simulink model "DC_DC"  (R2020b)
settings: Solver=VariableStepAuto  StartTime=0.0  StopTime=0.1  RelTol=1e-3
libraries: powerlib x20, powerlib_meascontrol x1
settings Model: Creator=huang  LastModifiedBy=huang
settings SolverCC: ZeroCrossAlgorithm=Adaptive
settings DebuggingCC: IgnoredZcDiagnostic=none

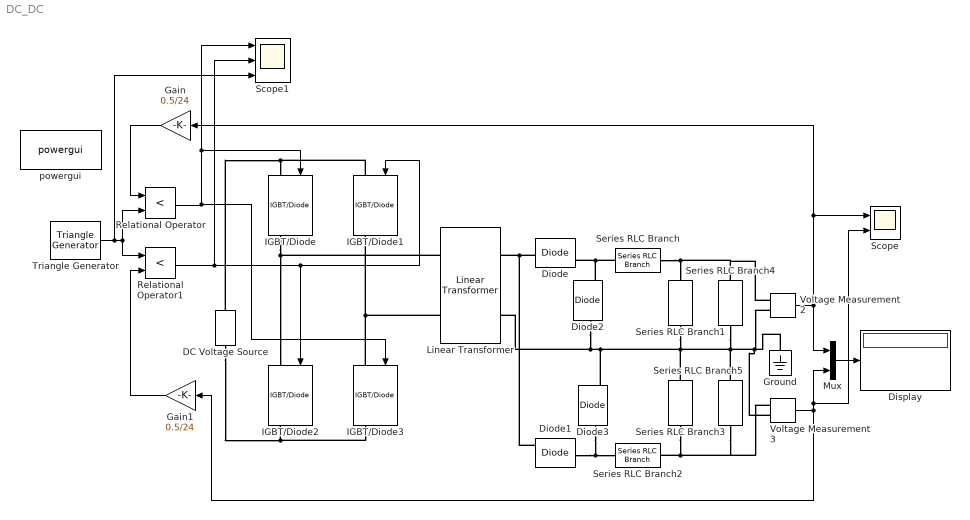
== system DC_DC ==
  DC Voltage Source : powerlib/Electrical Sources/DC Voltage Source  Amplitude=200  Measurements=None
  Diode{,1..3} (4 alike) : powerlib/Power Electronics/Diode  Ron=0.001  Lon=0  Vf=0.8  IC=0  UseSnubber=0  Rs=500  Cs=250e-9  Measurements=on
  Display : Display
  Gain : Gain  Gain=0.5/24
  Gain1 : Gain  Gain=0.5/24
  Ground : powerlib/Elements/Ground  LConnTagsString=a
  IGBT/Diode{,1..3} (4 alike) : powerlib/Power Electronics/IGBT//Diode  Ron=1e-3  Rs=1e5  Cs=inf  Measurements=on
  Linear Transformer : powerlib/Elements/Linear Transformer  UNITS=SI  NominalPower=[ 200 20e3 ]  winding1=[200 8e-08 5.0929e-11]  winding2=[48*2 2e-08 1.2732e-11]  ThreeWindings=off  winding3=[24*2 2e-08 1.2732e-11]  RmLm=[0.020001 3.1831e-07]  Measurements=None  DataType=on
  Mux : Mux  Inputs=2
  Relational Operator : RelationalOperator  Operator=<  OutDataTypeStr=boolean  RndMeth=Simplest
  Relational Operator1 : RelationalOperator  Operator=<  OutDataTypeStr=boolean  RndMeth=Simplest
  Scope : Scope  NumInputPorts=2
  Scope1 : Scope  NumInputPorts=3
  Series RLC Branch : powerlib/Elements/Series RLC Branch  LConnTagsString=__new0  RConnTagsString=__new0  BranchType=L  Resistance=1  Inductance=2e-3  SetiL0=off  InitialCurrent=0  Capacitance=1e-6  Setx0=off  InitialVoltage=0  Measurements=None
  Series RLC Branch1 : powerlib/Elements/Series RLC Branch  LConnTagsString=__new0  RConnTagsString=__new0  BranchType=C  Resistance=1  Inductance=1e-3  SetiL0=off  InitialCurrent=0  Capacitance=100e-6  Setx0=off  InitialVoltage=0  Measurements=None
  Series RLC Branch2 : powerlib/Elements/Series RLC Branch  LConnTagsString=__new0  RConnTagsString=__new0  BranchType=L  Resistance=1  Inductance=2e-3  SetiL0=off  InitialCurrent=0  Capacitance=1e-6  Setx0=off  InitialVoltage=0  Measurements=None
  Series RLC Branch3 : powerlib/Elements/Series RLC Branch  LConnTagsString=__new0  RConnTagsString=__new0  BranchType=C  Resistance=1  Inductance=1e-3  SetiL0=off  InitialCurrent=0  Capacitance=100e-6  Setx0=off  InitialVoltage=0  Measurements=None
  Series RLC Branch4 : powerlib/Elements/Series RLC Branch  LConnTagsString=__new0  RConnTagsString=__new0  BranchType=R  Resistance=24*24/200  Inductance=1e-3  SetiL0=off  InitialCurrent=0  Capacitance=100e-6  Setx0=off  InitialVoltage=0  Measurements=None
  Series RLC Branch5 : powerlib/Elements/Series RLC Branch  LConnTagsString=__new0  RConnTagsString=__new0  BranchType=R  Resistance=24*24/200  Inductance=1e-3  SetiL0=off  InitialCurrent=0  Capacitance=100e-6  Setx0=off  InitialVoltage=0  Measurements=None
  Triangle Generator : powerlib_meascontrol/Pulse & Signal Generators/Triangle Generator  Freq=20e3  Phase=90  Ts=0
  Voltage Measurement2 : powerlib/Measurements/Voltage Measurement  PhasorSimulation=off  OutputType=Complex  PSBequivalent=0
  Voltage Measurement3 : powerlib/Measurements/Voltage Measurement  PhasorSimulation=off  OutputType=Complex  PSBequivalent=0
  powergui : powerlib/powergui  Priority=1  SimulationMode=Continuous  SampleTime=50e-6  frequency=60  Iterations=50  frequencyindice=0  Pbase=100e6  ErrMax=1e-4  UnitsV=kV  UnitsW=MW  buscounter=0  FunctionMessages=off  echomessages=off  EnableUseOfTLC=off  CurrentSourceSwitches=off  DisableSnubberDevices=off  DisableRonSwitches=off  DisableVfSwitches=off  DisplayEquations=off  AutomaticDiscreteSolvers=off  SolverType=Tustin/Backward Euler (TBE)  Interpol=off  ExternalGateDelay=off  methode=off  Ts=100  x0status=blocks  SPID=on  SwTol=0  HookPort=off  NonlinearTolerance=1e-4  nMaxIteration=100  ContinueOnMaxIteration=off  RestoreLinks=warning  ResistiveCurrentMeasurement=off  Frange=[0:2:500]  Ylog=off  Xlog=on  ShowGrid=off  save=off  variable=ZData  structure=0  ZoomFFT=off  StartTime=0.0  cycles=1  DisplayStyle=1  fundamental=60  FreqAxis=off  MaxFrequency=1000  frequencyindicesteady=1  RmsSteady=1  display=off
  wires:
  Gain/1 -> Relational Operator/1
  Mux/1 -> Display/1
  Triangle Generator/1 -> Scope1/3, Relational Operator1/1, Relational Operator/2
  Gain1/1 -> Relational Operator1/2
  Relational Operator/1 -> IGBT/Diode3/1, Scope1/1, IGBT/Diode/1
  Relational Operator1/1 -> Scope1/2, IGBT/Diode2/1, IGBT/Diode1/1
  Voltage Measurement2/1 -> Mux/1, Gain/1, Scope/1
  Voltage Measurement3/1 -> Gain1/1, Scope/2, Mux/2
  connections:
  Diode/LConn1 -- Diode1/RConn1 -- Linear Transformer/RConn1
  Series RLC Branch/LConn1 -- Diode2/RConn1 -- Diode/RConn1
  Series RLC Branch/RConn1 -- Voltage Measurement2/LConn1 -- Series RLC Branch4/LConn1 -- Series RLC Branch1/LConn1
  Series RLC Branch1/RConn1 -- Ground/LConn1 -- Voltage Measurement2/LConn2 -- Voltage Measurement3/LConn2 -- Series RLC Branch5/LConn1 -- Series RLC Branch4/RConn1 -- Series RLC Branch3/LConn1 -- Diode3/RConn1 -- Diode2/LConn1 -- Linear Transformer/RConn2
  Series RLC Branch3/RConn1 -- Series RLC Branch5/RConn1 -- Voltage Measurement3/LConn1 -- Series RLC Branch2/RConn1
  Diode1/LConn1 -- Diode3/LConn1 -- Series RLC Branch2/LConn1
  IGBT/Diode3/LConn1 -- Linear Transformer/LConn2 -- IGBT/Diode1/RConn1
  IGBT/Diode/RConn1 -- Linear Transformer/LConn1 -- IGBT/Diode2/LConn1
  DC Voltage Source/RConn1 -- IGBT/Diode1/LConn1 -- IGBT/Diode/LConn1
  DC Voltage Source/LConn1 -- IGBT/Diode3/RConn1 -- IGBT/Diode2/RConn1
